simulink model "proj_baseline_tt"  (R2019b)
settings: Solver=VariableStepAuto  StartTime=0.0  StopTime=10.0  RelTol=1e-3
values from neighbouring files (symbols this model uses):
  Ac = [0, 1,                 0,              0 ... (first row only)    [model.m]    (also in proj_constants.m)
  Bc = [0;(I+m*l^2)/den; 0; m*l/den]    [model.m]    (also in proj_constants.m)
  Cc = [1 0 0 0 ... (first row only)    [model.m]    (also in proj_constants.m)
  Pq = 0.0000001 * eye(4)    [proj_constants.m]
  Pr = 0.0000001 * eye(2)    [proj_constants.m]
libraries: truetime x1
settings Model: Creator=jania  LastModifiedBy=jania

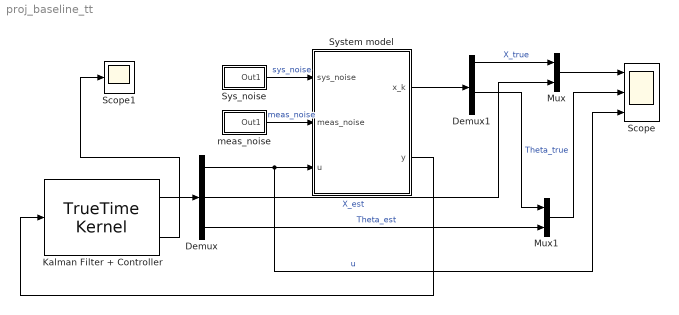
== system proj_baseline_tt ==
  Demux : Demux  Outputs=3
  Demux1 : Demux
  Kalman Filter + Controller : truetime/TrueTime Kernel  sfun=baseline_kernel_init  args=0.01  ninputsoutputs=[2 3]  ntriggers=0  trigtype=falling  nwnodenbr=[]  clockoffsetdrift=[0 0]  schedoutput=on  battery=off  poweroutput=off
  Mux : Mux  Inputs=2
  Mux1 : Mux  Inputs=2
  Scope : Scope  NumInputPorts=3
  Scope1 : Scope
  "Sys_noise " : Subsystem
  System model : Subsystem
  meas_noise : Subsystem
  wires:
  meas_noise/1(Out1) -> System model/2(meas_noise)  "meas_noise"
  "Sys_noise "/1(Out1) -> System model/1(sys_noise)  "sys_noise"
  Kalman Filter + Controller/1 -> Demux/1
  System model/2(y) -> Kalman Filter + Controller/1
  Demux/1 -> Scope/3, System model/3(u)  "u"
  System model/1(x_k) -> Demux1/1
  Mux/1 -> Scope/1
  Mux1/1 -> Scope/2
  Demux/3 -> Mux1/2  "Theta_est"
  Demux1/1 -> Mux/1  "X_true"
  Demux/2 -> Mux/2  "X_est"
  Demux1/3 -> Mux1/1  "Theta_true"
  Kalman Filter + Controller/2 -> Scope1/1

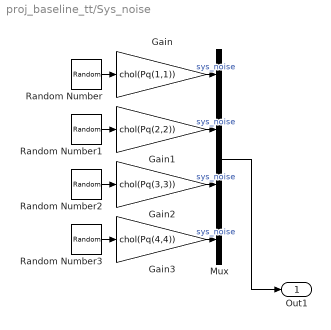
== system proj_baseline_tt/Sys_noise  ==
  Gain : Gain  Gain=chol(Pq(1,1))
  Gain1 : Gain  Gain=chol(Pq(2,2))
  Gain2 : Gain  Gain=chol(Pq(3,3))
  Gain3 : Gain  Gain=chol(Pq(4,4))
  Mux : Mux
  Random Number{,1..3} (4 alike) : RandomNumber
  Out1 : Outport
  wires:
  Gain2/1 -> Mux/3  "sys_noise"
  Random Number3/1 -> Gain3/1
  Gain1/1 -> Mux/2  "sys_noise"
  Gain3/1 -> Mux/4  "sys_noise"
  Random Number/1 -> Gain/1
  Mux/1 -> Out1/1
  Gain/1 -> Mux/1  "sys_noise"
  Random Number1/1 -> Gain1/1
  Random Number2/1 -> Gain2/1

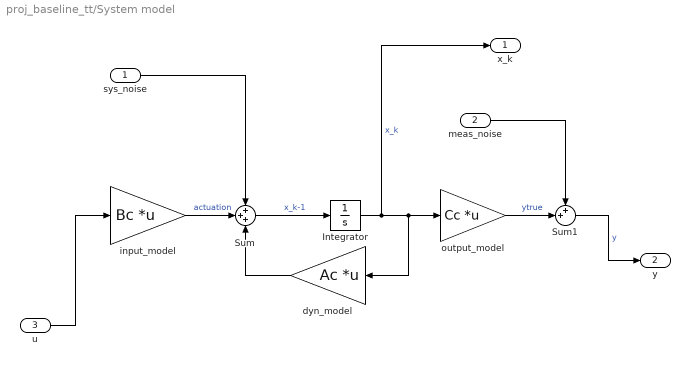
== system proj_baseline_tt/System model ==
  sys_noise : Inport
  meas_noise : Inport  Port=2
  u : Inport  Port=3
  Integrator : Integrator
  Sum : Sum  Inputs=+++
  Sum1 : Sum  Inputs=++|
  dyn_model : Gain  Gain=Ac  Multiplication=Matrix(K*u)
  input_model : Gain  Gain=Bc  Multiplication=Matrix(K*u)
  output_model : Gain  Gain=Cc  Multiplication=Matrix(K*u)
  x_k : Outport
  y : Outport  Port=2
  wires:
  Integrator/1 -> x_k/1, output_model/1, dyn_model/1  "x_k"
  Sum/1 -> Integrator/1  "x_k-1"
  meas_noise/1 -> Sum1/1
  input_model/1 -> Sum/2  "actuation"
  sys_noise/1 -> Sum/1
  dyn_model/1 -> Sum/3
  output_model/1 -> Sum1/2  "ytrue"
  u/1 -> input_model/1
  Sum1/1 -> y/1  "y"

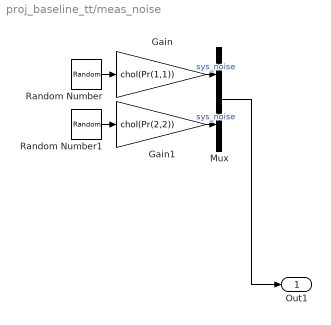
== system proj_baseline_tt/meas_noise ==
  Gain : Gain  Gain=chol(Pr(1,1))
  Gain1 : Gain  Gain=chol(Pr(2,2))
  Mux : Mux  Inputs=2
  Random Number : RandomNumber
  Random Number1 : RandomNumber
  Out1 : Outport
  wires:
  Gain1/1 -> Mux/2  "sys_noise"
  Random Number/1 -> Gain/1
  Mux/1 -> Out1/1
  Gain/1 -> Mux/1  "sys_noise"
  Random Number1/1 -> Gain1/1
